simulink model "influentgenerator_BSM"  (R2017a)
settings: Solver=ode45  StartTime=0  StopTime=365  RelTol=1e-6  AbsTol=1e-8  EnableMultiTasking=on
values from neighbouring files (symbols this model uses):
  amp = 0.05    [influentgeneratorinit.m]
  domestic_avg1 = [(1-codpart_frac1)*150/1000 codpart_frac1*150/1000  10/1000 15/1000 1.5/1000 QperPE1]    [influentgeneratorinit.m]
  emc_codsol = 9/1000    (= 0.009)    [influentgeneratorinit.m]
  emc_nh4 = 0.56/1000    (= 0.00056)    [influentgeneratorinit.m]
  evaporation_on = 1    [influentgeneratorinit.m]
  FFfraction1 = 0.25    [influentgeneratorinit.m]
  freq = 2*pi/365    (= 0.017214206321)    [influentgeneratorinit.m]
  gwbias1 = 95000    [influentgeneratorinit.m]
  imp_area1 = 250    [influentgeneratorinit.m]
  industrial_avg1 = [2000, 8000, 500, 800, 50, Qind_daily1]    [influentgeneratorinit.m]
  noise_std = 0.1    [influentgeneratorinit.m]
  pe1 = 400000    [influentgeneratorinit.m]
  perv_area1 = 1000    [influentgeneratorinit.m]
  phase = -3*pi/2    (= -4.71238898038)    [influentgeneratorinit.m]
  rrc1 = 1    [influentgeneratorinit.m]
  subareas1 = 7    [influentgeneratorinit.m]
  TAmp = 4    [influentgeneratorinit.m]
  TBias = 16    [influentgeneratorinit.m]
  TdAmp = 0.7    [influentgeneratorinit.m]
  TdBias = 0    [influentgeneratorinit.m]
  TdFreq = 2*pi    (= 6.28318530718)    [influentgeneratorinit.m]
  TdPhase = 0.25*pi    (= 0.785398163397)    [influentgeneratorinit.m]
  temp_correction = 2    [influentgeneratorinit.m]
  TFreq = freq    (= 0.017214206321)    [influentgeneratorinit.m]
  TPhase = -0.4*2*pi    (= -2.51327412287)    [influentgeneratorinit.m]
Description:
  | BSM2 influent model, version 15 March 2005
settings Model: SimulationMode=rapid-accelerator  ExtModeTrigDuration=100  Creator=Krist V. Gernaey  LastModifiedBy=ielsaagi
settings SolverCC: MaxConsecutiveMinStep=10
settings DataIOCC: SaveFinalState=on  SaveFormat=StructureWithTime  SignalLoggingSaveFormat=ModelDataLogs  SaveOutput=off  SaveState=on  DSMLogging=off  VisualizeSimOutput=off  SaveTime=off  StateSaveName=tmp_raccel_xout  SignalLoggingName=tmp_raccel_logsout  OutputOption=SpecifiedOutputTimes  OutputTimes=[0:1/(24*4):365]  Refine=5
settings OptimizationCC: BlockReduction=off  ExpressionDepthLimit=2147483647  InitFltsAndDblsToZero=on  EfficientMapNaN2IntZero=off  LifeSpan=inf  SimCompilerOptimization=on
settings DebuggingCC: ConsistencyChecking=warning  SaveWithParameterizedLinksMsg=none  UnderspecifiedInitializationDetection=Classic  MergeDetectMultiDrivingBlocksExec=none  MaxConsecutiveZCsMsg=warning  SolverPrmCheckMsg=warning  MultiTaskDSMMsg=warning  MultiTaskCondExecSysMsg=none  FcnCallInpInsideContextMsg=warning  ModelReferenceExtraNoncontSigs=warning  StateNameClashWarn=warning  SFUnexpectedBacktrackingDiag=warning  SFNoUnconditionalDefaultTransitionDiag=warning  SFExecutionAtInitializationDiag=none
settings HardwareCC: ProdBitPerPointer=32  ProdBitPerSizeT=32  ProdBitPerPtrDiffT=32  ProdLargestAtomicFloat=None  ProdIntDivRoundTo=Undefined  ProdEndianess=Unspecified  ProdWordSize=32  ProdHWDeviceType=32-bit Generic  TargetBitPerPointer=64  TargetBitPerSizeT=64  TargetBitPerPtrDiffT=64  TargetLongLongMode=on  TargetIntDivRoundTo=Zero  TargetEndianess=LittleEndian  TargetWordSize=64  TargetHWDeviceType=MATLAB Host  ProdEqTarget=off
settings ModelReferenceCC: PropagateSignalLabelsOutOfModel=off
settings SFSimCC: SFSimEcho=off
settings RTWCC: SystemTargetFile=raccel.tlc  TemplateMakefile=raccel_default_tmf  RTWVerbose=off  RTWUseSimCustomCode=on
settings CodeAppCC: GenerateComments=off  MaxIdLength=128  MangleLength=10  SimulinkBlockComments=off
settings RaccelTargetCC: GeneratePreprocessorConditionals=Use local settings  ERTFirstTimeCompliant=off  MultiInstanceERTCode=off  ENABLE_SLEXEC_SSBRIDGE=0  RTWCAPISignals=off  RTWCAPIParams=on
settings ConfigComp: CovMetricSettings=dw  CovHtmlReporting=on  CovSaveCumulativeToWorkspaceVar=on  CovSaveSingleToWorkspaceVar=on  CovExternalEMLEnable=off  CovSFcnEnable=off

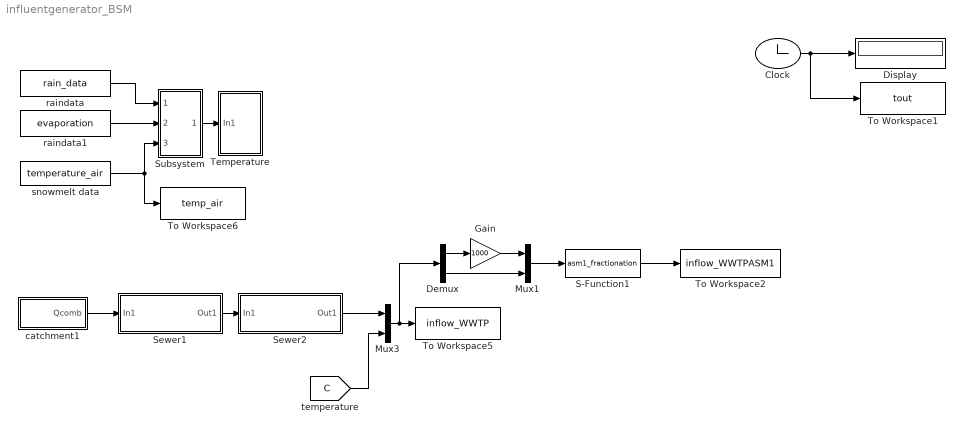
== system influentgenerator_BSM ==
  Clock : Clock
  Demux : Demux  Outputs=[5 2]
  Display : Display
  Gain : Gain  Gain=1000
  Mux1 : Mux  Inputs=2
  Mux3 : Mux  Inputs=2
  S-Function1 : S-Function  FunctionName=asm1_fractionation  Parameters=ASM1_FRACTIONS  SFunctionDeploymentMode=off  EnableBusSupport=off
  Sewer1 : Subsystem
  Sewer2 : Subsystem
  Subsystem : Subsystem
  Temperature : Subsystem
  To Workspace1 : ToWorkspace  VariableName=tout  SampleTime=-1
  To Workspace2 : ToWorkspace  VariableName=inflow_WWTPASM1  SampleTime=-1
  To Workspace5 : ToWorkspace  VariableName=inflow_WWTP  SampleTime=-1
  To Workspace6 : ToWorkspace  VariableName=temp_air  SampleTime=-1
  catchment1 : Subsystem
  raindata : FromWorkspace  VariableName=rain_data  OutDataTypeStr=double  SampleTime=0  Interpolate=off  OutputAfterFinalValue=Setting to zero
  raindata1 : FromWorkspace  VariableName=evaporation  OutDataTypeStr=double  SampleTime=30  Interpolate=off  OutputAfterFinalValue=Cyclic repetition
  snowmelt data : FromWorkspace  VariableName=temperature_air  SampleTime=0
  wires:
  Clock/1 -> To Workspace1/1, Display/1
  catchment1/1(Qcomb) -> Sewer1/1(In1)
  Sewer1/1(Out1) -> Sewer2/1(In1)
  Subsystem/1(Out1) -> Temperature/1(In1)
  raindata/1 -> Subsystem/1(In1)
  raindata1/1 -> Subsystem/2(In2)
  snowmelt data/1 -> To Workspace6/1, Subsystem/3(In3)
  [C] -> Mux3/2
  Sewer2/1(Out1) -> Mux3/1
  S-Function1/1 -> To Workspace2/1
  Mux1/1 -> S-Function1/1
  Demux/2 -> Mux1/2
  Gain/1 -> Mux1/1
  Mux3/1 -> Demux/1, To Workspace5/1
  Demux/1 -> Gain/1

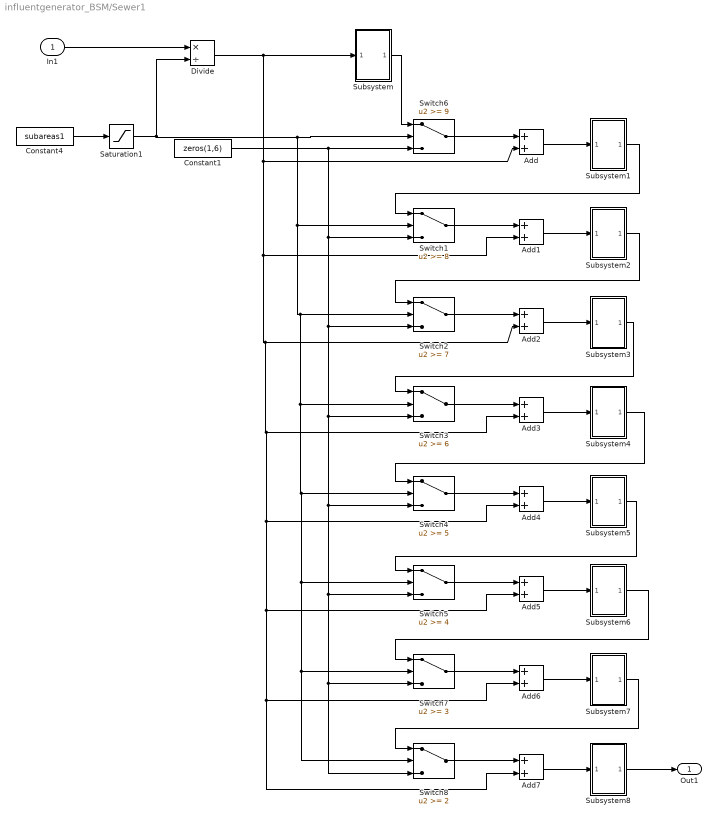
== system influentgenerator_BSM/Sewer1 ==
  In1 : Inport
  Add{,1..7} (8 alike) : Sum
  Constant1 : Constant  Value=zeros(1,6)
  Constant4 : Constant  Value=subareas1
  Divide : Product  Inputs=*/
  Saturation1 : Saturate  UpperLimit=9  LowerLimit=1
  Subsystem : Subsystem
  Subsystem1 : Subsystem
  Subsystem2 : Subsystem
  Subsystem3 : Subsystem
  Subsystem4 : Subsystem
  Subsystem5 : Subsystem
  Subsystem6 : Subsystem
  Subsystem7 : Subsystem
  Subsystem8 : Subsystem
  Switch1 : Switch  Threshold=8  SaturateOnIntegerOverflow=on
  Switch2 : Switch  Threshold=7  SaturateOnIntegerOverflow=on
  Switch3 : Switch  Threshold=6  SaturateOnIntegerOverflow=on
  Switch4 : Switch  Threshold=5  SaturateOnIntegerOverflow=on
  Switch5 : Switch  Threshold=4  SaturateOnIntegerOverflow=on
  Switch6 : Switch  Threshold=9  SaturateOnIntegerOverflow=on
  Switch7 : Switch  Threshold=3  SaturateOnIntegerOverflow=on
  Switch8 : Switch  Threshold=2  SaturateOnIntegerOverflow=on
  Out1 : Outport
  wires:
  In1/1 -> Divide/1
  Constant4/1 -> Saturation1/1
  Subsystem/1(Out1) -> Switch6/1
  Switch6/1 -> Add/1
  Add/1 -> Subsystem1/1(In1)
  Switch1/1 -> Add1/1
  Add1/1 -> Subsystem2/1(In1)
  Subsystem1/1(Out1) -> Switch1/1
  Subsystem2/1(Out1) -> Switch2/1
  Switch2/1 -> Add2/1
  Add2/1 -> Subsystem3/1(In1)
  Subsystem3/1(Out1) -> Switch3/1
  Add3/1 -> Subsystem4/1(In1)
  Switch3/1 -> Add3/1
  Subsystem4/1(Out1) -> Switch4/1
  Add4/1 -> Subsystem5/1(In1)
  Switch4/1 -> Add4/1
  Subsystem5/1(Out1) -> Switch5/1
  Add5/1 -> Subsystem6/1(In1)
  Switch5/1 -> Add5/1
  Subsystem6/1(Out1) -> Switch7/1
  Add6/1 -> Subsystem7/1(In1)
  Switch7/1 -> Add6/1
  Subsystem7/1(Out1) -> Switch8/1
  Add7/1 -> Subsystem8/1(In1)
  Switch8/1 -> Add7/1
  Saturation1/1 -> Divide/2, Switch8/2, Switch7/2, Switch5/2, Switch4/2, Switch3/2, Switch2/2, Switch1/2, Switch6/2
  Divide/1 -> Add6/2, Add7/2, Add5/2, Add4/2, Add3/2, Add2/2, Add1/2, Add/2, Subsystem/1(In1)
  Constant1/1 -> Switch8/3, Switch7/3, Switch5/3, Switch4/3, Switch3/3, Switch2/3, Switch1/3, Switch6/3
  Subsystem8/1(Out1) -> Out1/1

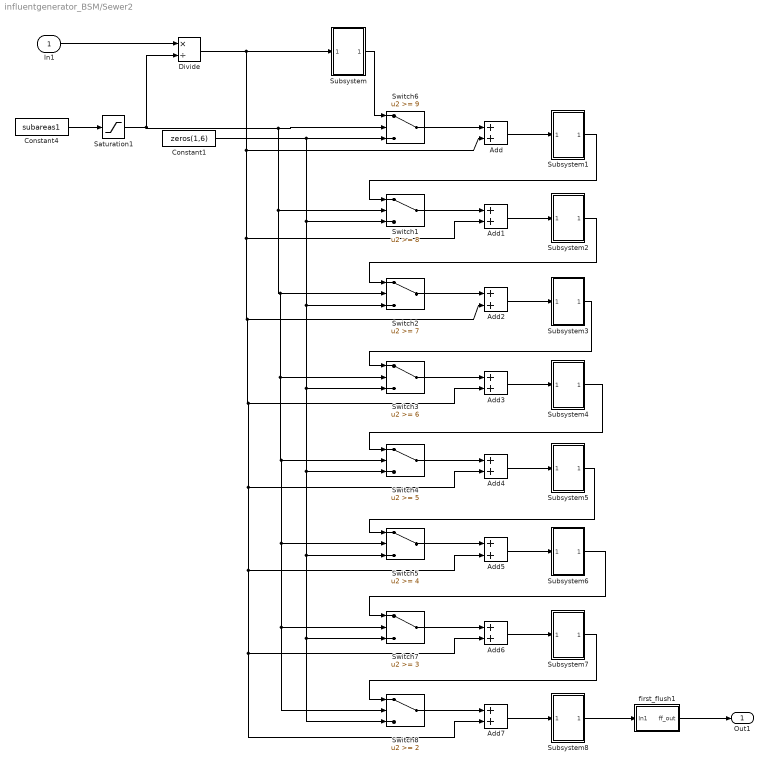
== system influentgenerator_BSM/Sewer2 ==
  In1 : Inport
  Add{,1..7} (8 alike) : Sum
  Constant1 : Constant  Value=zeros(1,6)
  Constant4 : Constant  Value=subareas1
  Divide : Product  Inputs=*/
  Saturation1 : Saturate  UpperLimit=9  LowerLimit=1
  Subsystem : Subsystem
  Subsystem1 : Subsystem
  Subsystem2 : Subsystem
  Subsystem3 : Subsystem
  Subsystem4 : Subsystem
  Subsystem5 : Subsystem
  Subsystem6 : Subsystem
  Subsystem7 : Subsystem
  Subsystem8 : Subsystem
  Switch1 : Switch  Threshold=8  SaturateOnIntegerOverflow=on
  Switch2 : Switch  Threshold=7  SaturateOnIntegerOverflow=on
  Switch3 : Switch  Threshold=6  SaturateOnIntegerOverflow=on
  Switch4 : Switch  Threshold=5  SaturateOnIntegerOverflow=on
  Switch5 : Switch  Threshold=4  SaturateOnIntegerOverflow=on
  Switch6 : Switch  Threshold=9  SaturateOnIntegerOverflow=on
  Switch7 : Switch  Threshold=3  SaturateOnIntegerOverflow=on
  Switch8 : Switch  Threshold=2  SaturateOnIntegerOverflow=on
  first_flush1 : Subsystem
  Out1 : Outport
  wires:
  In1/1 -> Divide/1
  Constant4/1 -> Saturation1/1
  Subsystem/1(Out1) -> Switch6/1
  Switch6/1 -> Add/1
  Add/1 -> Subsystem1/1(In1)
  Switch1/1 -> Add1/1
  Add1/1 -> Subsystem2/1(In1)
  Subsystem1/1(Out1) -> Switch1/1
  Subsystem2/1(Out1) -> Switch2/1
  Switch2/1 -> Add2/1
  Add2/1 -> Subsystem3/1(In1)
  Subsystem3/1(Out1) -> Switch3/1
  Add3/1 -> Subsystem4/1(In1)
  Switch3/1 -> Add3/1
  Subsystem4/1(Out1) -> Switch4/1
  Add4/1 -> Subsystem5/1(In1)
  Switch4/1 -> Add4/1
  Subsystem5/1(Out1) -> Switch5/1
  Add5/1 -> Subsystem6/1(In1)
  Switch5/1 -> Add5/1
  Subsystem6/1(Out1) -> Switch7/1
  Add6/1 -> Subsystem7/1(In1)
  Switch7/1 -> Add6/1
  Subsystem7/1(Out1) -> Switch8/1
  Add7/1 -> Subsystem8/1(In1)
  Switch8/1 -> Add7/1
  Saturation1/1 -> Divide/2, Switch8/2, Switch7/2, Switch5/2, Switch4/2, Switch3/2, Switch2/2, Switch1/2, Switch6/2
  Divide/1 -> Add6/2, Add7/2, Add5/2, Add4/2, Add3/2, Add2/2, Add1/2, Add/2, Subsystem/1(In1)
  Constant1/1 -> Switch8/3, Switch7/3, Switch5/3, Switch4/3, Switch3/3, Switch2/3, Switch1/3, Switch6/3
  first_flush1/1(ff_out) -> Out1/1
  Subsystem8/1(Out1) -> first_flush1/1(In1)

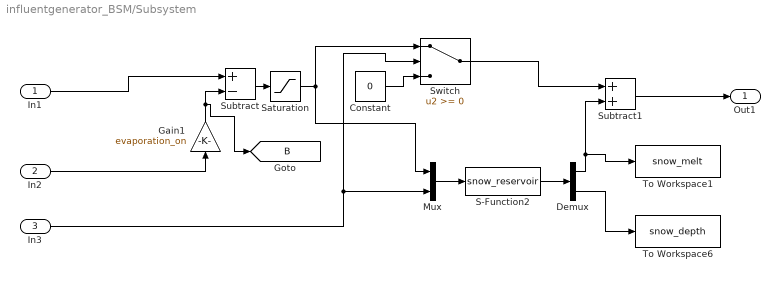
== system influentgenerator_BSM/Subsystem ==
  In1 : Inport
  In2 : Inport  Port=2
  In3 : Inport  Port=3
  Constant : Constant  Value=0
  Demux : Demux  Outputs=2
  Gain1 : Gain  Gain=evaporation_on
  Mux : Mux  Inputs=2
  S-Function2 : S-Function  FunctionName=snow_reservoir  Parameters=PAR_SNOW  SFunctionDeploymentMode=off  EnableBusSupport=off
  Saturation : Saturate  UpperLimit=inf  LowerLimit=0
  Subtract : Sum  Inputs=+-
  Subtract1 : Sum
  Switch : Switch
  To Workspace1 : ToWorkspace  VariableName=snow_melt  SampleTime=-1
  To Workspace6 : ToWorkspace  VariableName=snow_depth  SampleTime=-1
  Out1 : Outport
  tag scope: B=global
  wires:
  Demux/2 -> To Workspace6/1
  S-Function2/1 -> Demux/1
  In2/1 -> Gain1/1
  Subtract/1 -> Saturation/1
  Gain1/1 -> [B], Subtract/2
  Switch/1 -> Subtract1/1
  Constant/1 -> Switch/3
  Demux/1 -> To Workspace1/1, Subtract1/2
  Mux/1 -> S-Function2/1
  In3/1 -> Switch/2, Mux/2
  Subtract1/1 -> Out1/1
  Saturation/1 -> Mux/1, Switch/1
  In1/1 -> Subtract/1

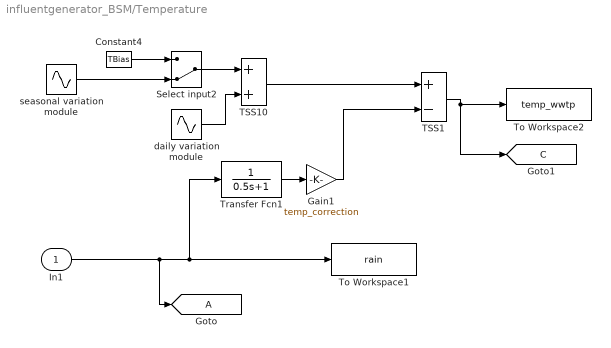
== system influentgenerator_BSM/Temperature ==
  In1 : Inport
  Constant4 : Constant  Value=TBias
  Gain1 : Gain  Gain=temp_correction
  Select input2 : ManualSwitch  CurrentSetting=0
  TSS1 : Sum  Inputs=+-
  TSS10 : Sum
  To Workspace1 : ToWorkspace  VariableName=rain  SampleTime=-1
  To Workspace2 : ToWorkspace  VariableName=temp_wwtp  SampleTime=-1
  Transfer Fcn1 : TransferFcn  Denominator=[0.5 1]
  daily variation module : Sin  Amplitude=TdAmp  Bias=TdBias  Frequency=TdFreq  Phase=TdPhase  SampleTime=0
  seasonal variation module : Sin  Amplitude=TAmp  Bias=TBias  Frequency=TFreq  Phase=TPhase  SampleTime=0
  tag scope: A=global, C=global
  wires:
  Select input2/1 -> TSS10/1
  Constant4/1 -> Select input2/1
  In1/1 -> Transfer Fcn1/1, To Workspace1/1, [A]
  TSS10/1 -> TSS1/1
  seasonal variation module/1 -> Select input2/2
  Transfer Fcn1/1 -> Gain1/1
  Gain1/1 -> TSS1/2
  daily variation module/1 -> TSS10/2
  TSS1/1 -> To Workspace2/1, [C]

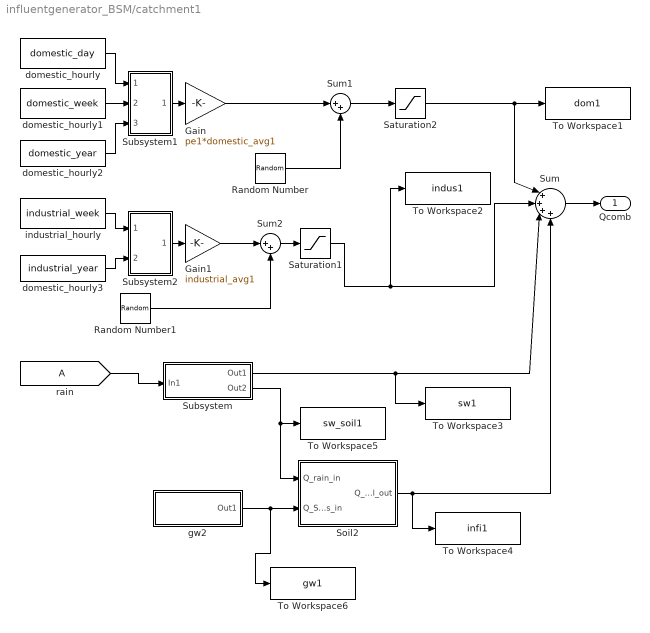
== system influentgenerator_BSM/catchment1 ==
  Gain : Gain  Gain=pe1*domestic_avg1  SampleTime=1/96
  Gain1 : Gain  Gain=industrial_avg1  SampleTime=1/96
  Random Number : RandomNumber  Variance=power(pe1*domestic_avg1*noise_std,2)  Seed=[7:1:12]  SampleTime=1/24
  Random Number1 : RandomNumber  Variance=power(industrial_avg1*noise_std,2)  Seed=[37:1:42]  SampleTime=1/24
  Saturation1 : Saturate  UpperLimit=industrial_avg1*10  LowerLimit=industrial_avg1*0
  Saturation2 : Saturate  UpperLimit=pe1*domestic_avg1*10  LowerLimit=pe1*domestic_avg1*0
  Soil2 : Subsystem
  Subsystem : Subsystem
  Subsystem1 : Subsystem
  Subsystem2 : Subsystem
  Sum : Sum  Inputs=|++++
  Sum1 : Sum  Inputs=|++
  Sum2 : Sum  Inputs=|++
  To Workspace1 : ToWorkspace  VariableName=dom1  SampleTime=-1
  To Workspace2 : ToWorkspace  VariableName=indus1  SampleTime=-1
  To Workspace3 : ToWorkspace  VariableName=sw1  SampleTime=-1
  To Workspace4 : ToWorkspace  VariableName=infi1  SampleTime=-1
  To Workspace5 : ToWorkspace  VariableName=sw_soil1  SampleTime=-1
  To Workspace6 : ToWorkspace  VariableName=gw1  SampleTime=-1
  domestic_hourly : FromWorkspace  VariableName=domestic_day  SampleTime=1/24  Interpolate=off  OutputAfterFinalValue=Cyclic repetition
  domestic_hourly1 : FromWorkspace  VariableName=domestic_week  SampleTime=1  Interpolate=off  OutputAfterFinalValue=Cyclic repetition
  domestic_hourly2 : FromWorkspace  VariableName=domestic_year  SampleTime=1  Interpolate=off  OutputAfterFinalValue=Cyclic repetition
  domestic_hourly3 : FromWorkspace  VariableName=industrial_year  SampleTime=1  Interpolate=off  OutputAfterFinalValue=Cyclic repetition
  gw2 : Subsystem
  industrial_hourly : FromWorkspace  VariableName=industrial_week  SampleTime=1/6  Interpolate=off  OutputAfterFinalValue=Cyclic repetition
  Qcomb : Outport
  wires:
  [A] -> Subsystem/1(In1)
  Sum1/1 -> Saturation2/1
  Sum2/1 -> Saturation1/1
  Subsystem/1(Out1) -> Sum/3, To Workspace3/1
  Sum/1 -> Qcomb/1
  domestic_hourly/1 -> Subsystem1/1(In1)
  domestic_hourly1/1 -> Subsystem1/2(In2)
  domestic_hourly2/1 -> Subsystem1/3(In3)
  Subsystem1/1(Out1) -> Gain/1
  domestic_hourly3/1 -> Subsystem2/2(In2)
  industrial_hourly/1 -> Subsystem2/1(In1)
  Subsystem2/1(Out1) -> Gain1/1
  Gain1/1 -> Sum2/1
  Random Number/1 -> Sum1/2
  Random Number1/1 -> Sum2/2
  Subsystem/2(Out2) -> To Workspace5/1, Soil2/1(Q_rain_in)
  gw2/1(Out1) -> To Workspace6/1, Soil2/2(Q_Seas_in)
  Soil2/1(Q_Soil_out) -> Sum/4, To Workspace4/1
  Saturation2/1 -> Sum/1, To Workspace1/1
  Saturation1/1 -> To Workspace2/1, Sum/2
  Gain/1 -> Sum1/1

== system influentgenerator_BSM/Sewer1/Subsystem ==
  In1 : Inport
  S-Function{1..3,15} (4 alike) : S-Function  FunctionName=reservoir  Parameters=PAR_RESERVOIR  SFunctionDeploymentMode=off  EnableBusSupport=off
  Out1 : Outport
  wires:
  S-Function3/1 -> Out1/1
  S-Function1/1 -> S-Function2/1
  S-Function2/1 -> S-Function3/1
  In1/1 -> S-Function15/1
  S-Function15/1 -> S-Function1/1

== system influentgenerator_BSM/Sewer1/Subsystem1 ==
  In1 : Inport
  S-Function{1..3,15} (4 alike) : S-Function  FunctionName=reservoir  Parameters=PAR_RESERVOIR  SFunctionDeploymentMode=off  EnableBusSupport=off
  Out1 : Outport
  wires:
  S-Function3/1 -> Out1/1
  S-Function1/1 -> S-Function2/1
  S-Function2/1 -> S-Function3/1
  In1/1 -> S-Function15/1
  S-Function15/1 -> S-Function1/1

== system influentgenerator_BSM/Sewer1/Subsystem2 ==
  In1 : Inport
  S-Function{1..3,15} (4 alike) : S-Function  FunctionName=reservoir  Parameters=PAR_RESERVOIR  SFunctionDeploymentMode=off  EnableBusSupport=off
  Out1 : Outport
  wires:
  S-Function3/1 -> Out1/1
  S-Function1/1 -> S-Function2/1
  S-Function2/1 -> S-Function3/1
  In1/1 -> S-Function15/1
  S-Function15/1 -> S-Function1/1

== system influentgenerator_BSM/Sewer1/Subsystem3 ==
  In1 : Inport
  S-Function{1..3,15} (4 alike) : S-Function  FunctionName=reservoir  Parameters=PAR_RESERVOIR  SFunctionDeploymentMode=off  EnableBusSupport=off
  Out1 : Outport
  wires:
  S-Function3/1 -> Out1/1
  S-Function1/1 -> S-Function2/1
  S-Function2/1 -> S-Function3/1
  In1/1 -> S-Function15/1
  S-Function15/1 -> S-Function1/1

== system influentgenerator_BSM/Sewer1/Subsystem4 ==
  In1 : Inport
  S-Function{1..3,15} (4 alike) : S-Function  FunctionName=reservoir  Parameters=PAR_RESERVOIR  SFunctionDeploymentMode=off  EnableBusSupport=off
  Out1 : Outport
  wires:
  S-Function3/1 -> Out1/1
  S-Function1/1 -> S-Function2/1
  S-Function2/1 -> S-Function3/1
  In1/1 -> S-Function15/1
  S-Function15/1 -> S-Function1/1

== system influentgenerator_BSM/Sewer1/Subsystem5 ==
  In1 : Inport
  S-Function{1..3,15} (4 alike) : S-Function  FunctionName=reservoir  Parameters=PAR_RESERVOIR  SFunctionDeploymentMode=off  EnableBusSupport=off
  Out1 : Outport
  wires:
  S-Function3/1 -> Out1/1
  S-Function1/1 -> S-Function2/1
  S-Function2/1 -> S-Function3/1
  In1/1 -> S-Function15/1
  S-Function15/1 -> S-Function1/1

== system influentgenerator_BSM/Sewer1/Subsystem6 ==
  In1 : Inport
  S-Function{1..3,15} (4 alike) : S-Function  FunctionName=reservoir  Parameters=PAR_RESERVOIR  SFunctionDeploymentMode=off  EnableBusSupport=off
  Out1 : Outport
  wires:
  S-Function3/1 -> Out1/1
  S-Function1/1 -> S-Function2/1
  S-Function2/1 -> S-Function3/1
  In1/1 -> S-Function15/1
  S-Function15/1 -> S-Function1/1

== system influentgenerator_BSM/Sewer1/Subsystem7 ==
  In1 : Inport
  S-Function{1..3,15} (4 alike) : S-Function  FunctionName=reservoir  Parameters=PAR_RESERVOIR  SFunctionDeploymentMode=off  EnableBusSupport=off
  Out1 : Outport
  wires:
  S-Function3/1 -> Out1/1
  S-Function1/1 -> S-Function2/1
  S-Function2/1 -> S-Function3/1
  In1/1 -> S-Function15/1
  S-Function15/1 -> S-Function1/1

== system influentgenerator_BSM/Sewer1/Subsystem8 ==
  In1 : Inport
  S-Function{1..3,15} (4 alike) : S-Function  FunctionName=reservoir  Parameters=PAR_RESERVOIR  SFunctionDeploymentMode=off  EnableBusSupport=off
  Out1 : Outport
  wires:
  S-Function3/1 -> Out1/1
  S-Function1/1 -> S-Function2/1
  S-Function2/1 -> S-Function3/1
  In1/1 -> S-Function15/1
  S-Function15/1 -> S-Function1/1

== system influentgenerator_BSM/Sewer2/Subsystem ==
  In1 : Inport
  S-Function{1..3,15} (4 alike) : S-Function  FunctionName=reservoir  Parameters=PAR_RESERVOIR  SFunctionDeploymentMode=off  EnableBusSupport=off
  Out1 : Outport
  wires:
  S-Function3/1 -> Out1/1
  S-Function1/1 -> S-Function2/1
  S-Function2/1 -> S-Function3/1
  In1/1 -> S-Function15/1
  S-Function15/1 -> S-Function1/1

== system influentgenerator_BSM/Sewer2/Subsystem1 ==
  In1 : Inport
  S-Function{1..3,15} (4 alike) : S-Function  FunctionName=reservoir  Parameters=PAR_RESERVOIR  SFunctionDeploymentMode=off  EnableBusSupport=off
  Out1 : Outport
  wires:
  S-Function3/1 -> Out1/1
  S-Function1/1 -> S-Function2/1
  S-Function2/1 -> S-Function3/1
  In1/1 -> S-Function15/1
  S-Function15/1 -> S-Function1/1

== system influentgenerator_BSM/Sewer2/Subsystem2 ==
  In1 : Inport
  S-Function{1..3,15} (4 alike) : S-Function  FunctionName=reservoir  Parameters=PAR_RESERVOIR  SFunctionDeploymentMode=off  EnableBusSupport=off
  Out1 : Outport
  wires:
  S-Function3/1 -> Out1/1
  S-Function1/1 -> S-Function2/1
  S-Function2/1 -> S-Function3/1
  In1/1 -> S-Function15/1
  S-Function15/1 -> S-Function1/1

== system influentgenerator_BSM/Sewer2/Subsystem3 ==
  In1 : Inport
  S-Function{1..3,15} (4 alike) : S-Function  FunctionName=reservoir  Parameters=PAR_RESERVOIR  SFunctionDeploymentMode=off  EnableBusSupport=off
  Out1 : Outport
  wires:
  S-Function3/1 -> Out1/1
  S-Function1/1 -> S-Function2/1
  S-Function2/1 -> S-Function3/1
  In1/1 -> S-Function15/1
  S-Function15/1 -> S-Function1/1

== system influentgenerator_BSM/Sewer2/Subsystem4 ==
  In1 : Inport
  S-Function{1..3,15} (4 alike) : S-Function  FunctionName=reservoir  Parameters=PAR_RESERVOIR  SFunctionDeploymentMode=off  EnableBusSupport=off
  Out1 : Outport
  wires:
  S-Function3/1 -> Out1/1
  S-Function1/1 -> S-Function2/1
  S-Function2/1 -> S-Function3/1
  In1/1 -> S-Function15/1
  S-Function15/1 -> S-Function1/1

== system influentgenerator_BSM/Sewer2/Subsystem5 ==
  In1 : Inport
  S-Function{1..3,15} (4 alike) : S-Function  FunctionName=reservoir  Parameters=PAR_RESERVOIR  SFunctionDeploymentMode=off  EnableBusSupport=off
  Out1 : Outport
  wires:
  S-Function3/1 -> Out1/1
  S-Function1/1 -> S-Function2/1
  S-Function2/1 -> S-Function3/1
  In1/1 -> S-Function15/1
  S-Function15/1 -> S-Function1/1

== system influentgenerator_BSM/Sewer2/Subsystem6 ==
  In1 : Inport
  S-Function{1..3,15} (4 alike) : S-Function  FunctionName=reservoir  Parameters=PAR_RESERVOIR  SFunctionDeploymentMode=off  EnableBusSupport=off
  Out1 : Outport
  wires:
  S-Function3/1 -> Out1/1
  S-Function1/1 -> S-Function2/1
  S-Function2/1 -> S-Function3/1
  In1/1 -> S-Function15/1
  S-Function15/1 -> S-Function1/1

== system influentgenerator_BSM/Sewer2/Subsystem7 ==
  In1 : Inport
  S-Function{1..3,15} (4 alike) : S-Function  FunctionName=reservoir  Parameters=PAR_RESERVOIR  SFunctionDeploymentMode=off  EnableBusSupport=off
  Out1 : Outport
  wires:
  S-Function3/1 -> Out1/1
  S-Function1/1 -> S-Function2/1
  S-Function2/1 -> S-Function3/1
  In1/1 -> S-Function15/1
  S-Function15/1 -> S-Function1/1

== system influentgenerator_BSM/Sewer2/Subsystem8 ==
  In1 : Inport
  S-Function{1..3,15} (4 alike) : S-Function  FunctionName=reservoir  Parameters=PAR_RESERVOIR  SFunctionDeploymentMode=off  EnableBusSupport=off
  Out1 : Outport
  wires:
  S-Function3/1 -> Out1/1
  S-Function1/1 -> S-Function2/1
  S-Function2/1 -> S-Function3/1
  In1/1 -> S-Function15/1
  S-Function15/1 -> S-Function1/1

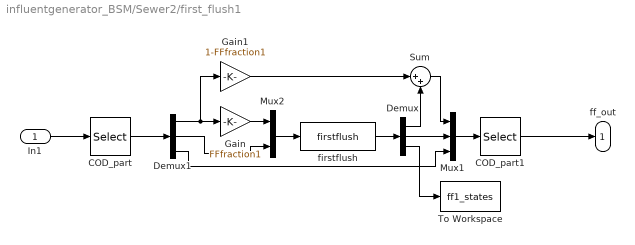
== system influentgenerator_BSM/Sewer2/first_flush1 ==
  In1 : Inport
  COD_part : Selector  InputPortWidth=6  IndexOptions=Index vector (dialog)  Indices=[2 6 1 3 4 5]  OutputSizes=1
  COD_part1 : Selector  InputPortWidth=6  IndexOptions=Index vector (dialog)  Indices=[3 1 4 5 6 2]  OutputSizes=1
  Demux : Demux  Outputs=[1 1 2]
  Demux1 : Demux  Outputs=[1 1 4]
  Gain : Gain  Gain=FFfraction1
  Gain1 : Gain  Gain=1-FFfraction1
  Mux1 : Mux  Inputs=3
  Mux2 : Mux  Inputs=2
  Sum : Sum  Inputs=|++
  To Workspace : ToWorkspace  VariableName=ff1_states  SampleTime=-1
  firstflush : S-Function  FunctionName=firstflush  Parameters=PAR_FIRSTFLUSH1  SFunctionDeploymentMode=off  EnableBusSupport=off
  ff_out : Outport
  wires:
  COD_part1/1 -> ff_out/1
  Mux2/1 -> firstflush/1
  In1/1 -> COD_part/1
  Gain/1 -> Mux2/1
  Demux/1 -> Sum/2
  Gain1/1 -> Sum/1
  COD_part/1 -> Demux1/1
  Demux1/1 -> Gain1/1, Gain/1
  Demux/2 -> Mux1/2
  Sum/1 -> Mux1/1
  Mux1/1 -> COD_part1/1
  Demux1/3 -> Mux1/3
  firstflush/1 -> Demux/1
  Demux1/2 -> Mux2/2
  Demux/3 -> To Workspace/1

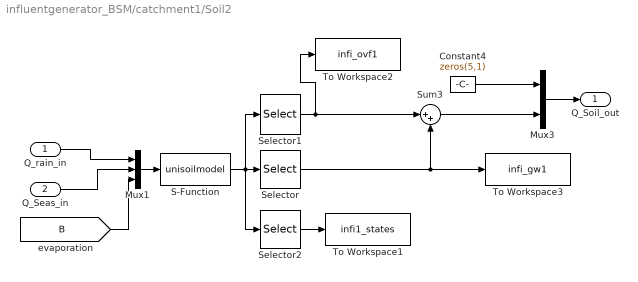
== system influentgenerator_BSM/catchment1/Soil2 ==
  Q_rain_in : Inport
  Q_Seas_in : Inport  Port=2
  Constant4 : Constant  Value=zeros(5,1)
  Mux1 : Mux  Inputs=3
  Mux3 : Mux  Inputs=2
  S-Function : S-Function  FunctionName=unisoilmodel  Parameters=XINITSOIL1, PARS_SOIL1  SFunctionDeploymentMode=off  EnableBusSupport=off
  Selector : Selector  InputPortWidth=4  IndexOptions=Index vector (dialog)  Indices=[1]  OutputSizes=1
  Selector1 : Selector  InputPortWidth=4  IndexOptions=Index vector (dialog)  Indices=[2]  OutputSizes=1
  Selector2 : Selector  InputPortWidth=4  IndexOptions=Index vector (dialog)  Indices=[4]  OutputSizes=1
  Sum3 : Sum  Inputs=|++  SaturateOnIntegerOverflow=on
  To Workspace1 : ToWorkspace  VariableName=infi1_states  SampleTime=-1
  To Workspace2 : ToWorkspace  VariableName=infi_ovf1  SampleTime=-1
  To Workspace3 : ToWorkspace  VariableName=infi_gw1  SampleTime=-1
  Q_Soil_out : Outport
  wires:
  Selector/1 -> To Workspace3/1, Sum3/2
  Mux1/1 -> S-Function/1
  Q_rain_in/1 -> Mux1/1
  Constant4/1 -> Mux3/1
  Sum3/1 -> Mux3/2
  Mux3/1 -> Q_Soil_out/1
  Q_Seas_in/1 -> Mux1/2
  S-Function/1 -> Selector2/1, Selector/1, Selector1/1
  Selector2/1 -> To Workspace1/1
  Selector1/1 -> Sum3/1, To Workspace2/1
  [B] -> Mux1/3

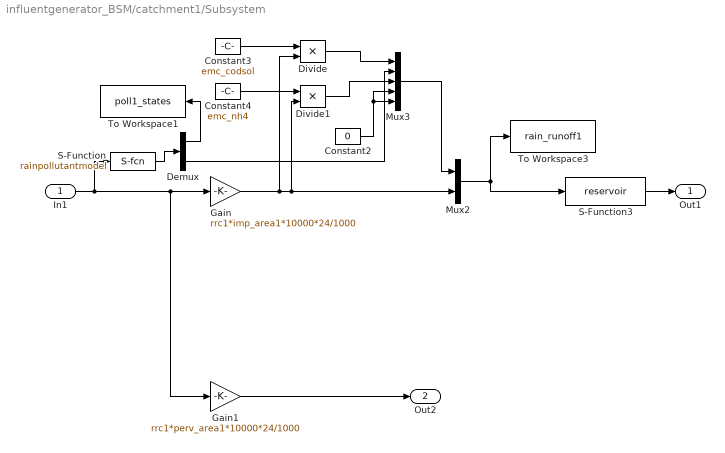
== system influentgenerator_BSM/catchment1/Subsystem ==
  In1 : Inport
  Constant2 : Constant  Value=0
  Constant3 : Constant  Value=emc_codsol
  Constant4 : Constant  Value=emc_nh4
  Demux : Demux  Outputs=2
  Divide : Product  Inputs=**
  Divide1 : Product  Inputs=**
  Gain : Gain  Gain=rrc1*imp_area1*10000*24/1000
  Gain1 : Gain  Gain=rrc1*perv_area1*10000*24/1000
  Mux2 : Mux  Inputs=2
  Mux3 : Mux  Inputs=5
  S-Function : S-Function  FunctionName=rainpollutantmodel  Parameters=PAR_QUALITY1, XINIT_QUALITY1  SFunctionDeploymentMode=off  EnableBusSupport=off
  S-Function3 : S-Function  FunctionName=reservoir  Parameters=PAR_RESERVOIR_rain  SFunctionDeploymentMode=off  EnableBusSupport=off
  To Workspace1 : ToWorkspace  VariableName=poll1_states  SampleTime=-1
  To Workspace3 : ToWorkspace  VariableName=rain_runoff1  SampleTime=-1
  Out1 : Outport
  Out2 : Outport  Port=2
  wires:
  In1/1 -> S-Function/1, Gain1/1, Gain/1
  Gain/1 -> Divide/2, Divide1/2, Mux2/2
  Constant2/1 -> Mux3/4, Mux3/5
  Mux3/1 -> Mux2/1
  Demux/2 -> Mux3/2
  Constant3/1 -> Divide/1
  Constant4/1 -> Divide1/1
  Divide/1 -> Mux3/1
  Divide1/1 -> Mux3/3
  S-Function3/1 -> Out1/1
  S-Function/1 -> Demux/1
  Demux/1 -> To Workspace1/1
  Mux2/1 -> S-Function3/1, To Workspace3/1
  Gain1/1 -> Out2/1

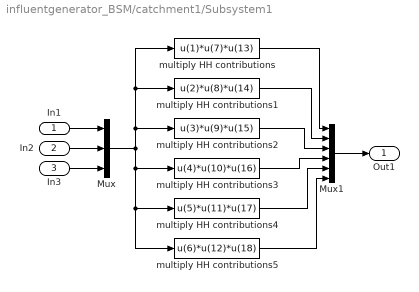
== system influentgenerator_BSM/catchment1/Subsystem1 ==
  In1 : Inport
  In2 : Inport  Port=2
  In3 : Inport  Port=3
  Mux : Mux  Inputs=3
  Mux1 : Mux  Inputs=6
  multiply HH contributions : Fcn  Expr=u(1)*u(7)*u(13)
  multiply HH contributions1 : Fcn  Expr=u(2)*u(8)*u(14)
  multiply HH contributions2 : Fcn  Expr=u(3)*u(9)*u(15)
  multiply HH contributions3 : Fcn  Expr=u(4)*u(10)*u(16)
  multiply HH contributions4 : Fcn  Expr=u(5)*u(11)*u(17)
  multiply HH contributions5 : Fcn  Expr=u(6)*u(12)*u(18)
  Out1 : Outport
  wires:
  In1/1 -> Mux/1
  In3/1 -> Mux/3
  In2/1 -> Mux/2
  Mux/1 -> multiply HH contributions3/1, multiply HH contributions4/1, multiply HH contributions5/1, multiply HH contributions2/1, multiply HH contributions1/1, multiply HH contributions/1
  multiply HH contributions/1 -> Mux1/1
  multiply HH contributions1/1 -> Mux1/2
  multiply HH contributions2/1 -> Mux1/3
  multiply HH contributions3/1 -> Mux1/4
  multiply HH contributions4/1 -> Mux1/5
  multiply HH contributions5/1 -> Mux1/6
  Mux1/1 -> Out1/1

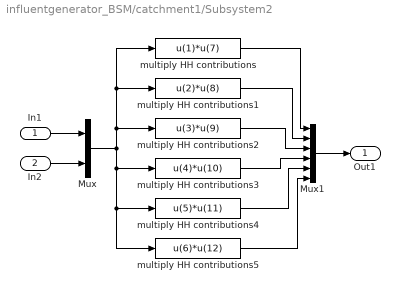
== system influentgenerator_BSM/catchment1/Subsystem2 ==
  In1 : Inport
  In2 : Inport  Port=2
  Mux : Mux  Inputs=2
  Mux1 : Mux  Inputs=6
  multiply HH contributions : Fcn  Expr=u(1)*u(7)
  multiply HH contributions1 : Fcn  Expr=u(2)*u(8)
  multiply HH contributions2 : Fcn  Expr=u(3)*u(9)
  multiply HH contributions3 : Fcn  Expr=u(4)*u(10)
  multiply HH contributions4 : Fcn  Expr=u(5)*u(11)
  multiply HH contributions5 : Fcn  Expr=u(6)*u(12)
  Out1 : Outport
  wires:
  In1/1 -> Mux/1
  In2/1 -> Mux/2
  Mux/1 -> multiply HH contributions3/1, multiply HH contributions4/1, multiply HH contributions5/1, multiply HH contributions2/1, multiply HH contributions1/1, multiply HH contributions/1
  multiply HH contributions/1 -> Mux1/1
  multiply HH contributions1/1 -> Mux1/2
  multiply HH contributions2/1 -> Mux1/3
  multiply HH contributions3/1 -> Mux1/4
  multiply HH contributions4/1 -> Mux1/5
  multiply HH contributions5/1 -> Mux1/6
  Mux1/1 -> Out1/1

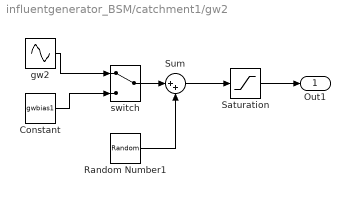
== system influentgenerator_BSM/catchment1/gw2 ==
  Constant : Constant  Value=gwbias1
  Random Number1 : RandomNumber  Variance=power(gwbias1*noise_std,2)  Seed=44  SampleTime=1/96
  Saturation : Saturate  UpperLimit=gwbias1*5  LowerLimit=0
  Sum : Sum  Inputs=|++
  gw2 : Sin  Amplitude=gwbias1*amp  Bias=gwbias1  Frequency=freq  Phase=phase  SampleTime=0
  "switch " : ManualSwitch
  Out1 : Outport
  wires:
  Random Number1/1 -> Sum/2
  gw2/1 -> "switch "/1
  Constant/1 -> "switch "/2
  Saturation/1 -> Out1/1
  "switch "/1 -> Sum/1
  Sum/1 -> Saturation/1
